simulink model "d_7_11_6"  (R2025a)
settings: Solver=VariableStepAuto  StartTime=0.0  StopTime=200  RelTol=1e-3
settings Model: Creator=Korisnik  LastModifiedBy=Korisnik

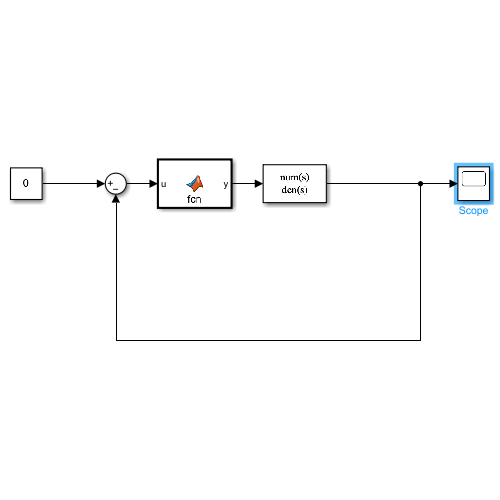
[thumbnail: Simulink's stored preview of the top-level diagram]
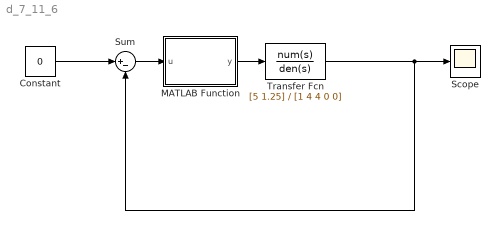
== system d_7_11_6 ==
  Constant : Constant  Value=0
  MATLAB Function : MATLAB Function  TreatAsAtomicUnit=on
  Scope : Scope
      settings: ActiveDisplayYMinimum=-3.8250737726049175  ActiveDisplayYMaximum=4.1548477444231313
  Sum : Sum  Inputs=|+-
  Transfer Fcn : TransferFcn  Numerator=[5 1.25]  Denominator=[1 4 4 0 0]
  wires:
  Transfer Fcn/1 -> Sum/2, Scope/1
  Constant/1 -> Sum/1
  Sum/1 -> MATLAB Function/1(u)
  MATLAB Function/1(y) -> Transfer Fcn/1

== matlab function d_7_11_6/MATLAB Function ==
  data: u input; y output
function y = fcn(u)
if u >= 0
    y = 2*u + 1;
else
    y = 2*u - 1;
end
end
